simulink model "plantFunction"  (R2024a)
settings: Solver=VariableStepAuto  StartTime=0.0  StopTime=10.0  RelTol=1e-3
settings Model: Creator=tn212  LastModifiedBy=tn212

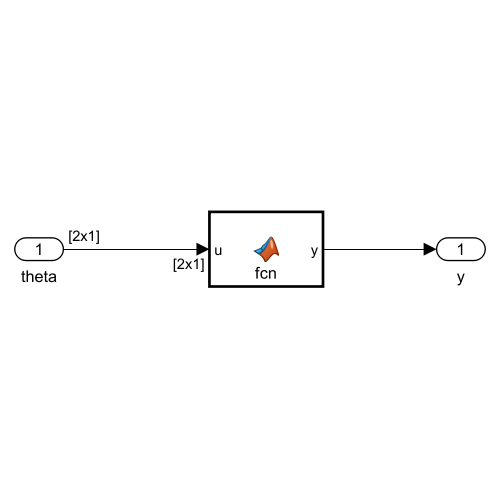
[thumbnail: Simulink's stored preview of the top-level diagram]
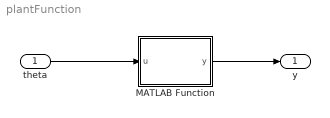
== system plantFunction ==
  theta : Inport  PortDimensions=[2 1]
  MATLAB Function : MATLAB Function  TreatAsAtomicUnit=on
  y : Outport
  wires:
  theta/1 -> MATLAB Function/1(u)
  MATLAB Function/1(y) -> y/1

== matlab function plantFunction/MATLAB Function ==
  data: u input; y output
function y = fcn(u)

y = -u(1)^2 - (u(2) - 1)^2;
